simulink model "ChkPwrMding_newLogic"  (Simulink 7.8)
settings: Solver=ode45  StartTime=0.0  StopTime=10.0  RelTol=1e-3
undefined symbols (not defined in the file): CeSTMR_e_LVR_N, CeSTMR_e_LVR_P, KeASMR_b_CheckParkAndNeutral, KeASMR_b_StrtCntrlOffChkEnbl
libraries: ChryslerLib x2
settings Model: Creator=Ben  LastModifiedBy=Ben

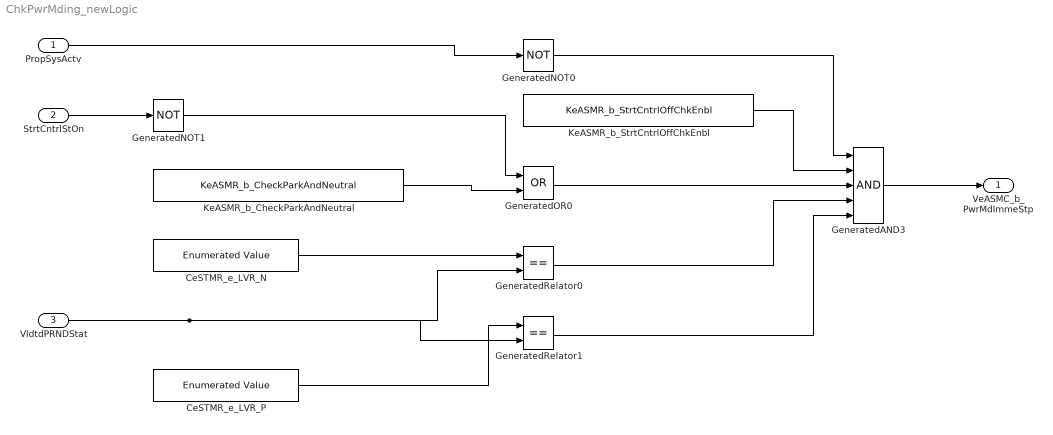
== system ChkPwrMding_newLogic ==
  PropSysActv : Inport
  StrtCntrlStOn : Inport  Port=2
  VldtdPRNDStat : Inport  Port=3
  CeSTMR_e_LVR_N : ChryslerLib/Parameters & Constants/Enumerated Value  Value=CeSTMR_e_LVR_N  OutMin=[]  OutMax=[]  OutDataTypeStr=TeSTMR_e_Lv2PRND_Stat
  CeSTMR_e_LVR_P : ChryslerLib/Parameters & Constants/Enumerated Value  Value=CeSTMR_e_LVR_P  OutMin=[]  OutMax=[]  OutDataTypeStr=TeSTMR_e_Lv2PRND_Stat
  GeneratedAND3 : Logic  Inputs=5
  GeneratedNOT0 : Logic  Operator=NOT
  GeneratedNOT1 : Logic  Operator=NOT
  GeneratedOR0 : Logic  Operator=OR
  GeneratedRelator0 : RelationalOperator  Operator===  InputSameDT=on
  GeneratedRelator1 : RelationalOperator  Operator===  InputSameDT=on
  KeASMR_b_CheckParkAndNeutral : Constant  Value=KeASMR_b_CheckParkAndNeutral
      settings: CopyFcn=try,set_param(gcb,'Value',get_param(gcb,'Name'));catch,err=lasterror;if (isempty(strfind(err.message,'Attempting to override parameters')) || isempty(strfind(err.message,'which is inside a library link'))) rethrow(err);end;end  NameChangeFcn=try,set_param(gcb,'Value',get_param(gcb,'Name'));catch,[msgstr msgid]=lasterr;errordlg(['error ',num2str(msgid),' - ',msgstr],'Error','modal');end  OpenFcn=global edelemcal; edelemcal.cb = gcb; edfigelemcal('fig');
  KeASMR_b_StrtCntrlOffChkEnbl : Constant  Value=KeASMR_b_StrtCntrlOffChkEnbl
      settings: CopyFcn=try,set_param(gcb,'Value',get_param(gcb,'Name'));catch,err=lasterror;if (isempty(strfind(err.message,'Attempting to override parameters')) || isempty(strfind(err.message,'which is inside a library link'))) rethrow(err);end;end  NameChangeFcn=try,set_param(gcb,'Value',get_param(gcb,'Name'));catch,[msgstr msgid]=lasterr;errordlg(['error ',num2str(msgid),' - ',msgstr],'Error','modal');end  OpenFcn=global edelemcal; edelemcal.cb = gcb; edfigelemcal('fig');
  VeASMC_b_PwrMdImmeStp : Outport
  wires:
  VldtdPRNDStat/1 -> GeneratedRelator0/2, GeneratedRelator1/2
  GeneratedNOT0/1 -> GeneratedAND3/1
  KeASMR_b_StrtCntrlOffChkEnbl/1 -> GeneratedAND3/2
  GeneratedOR0/1 -> GeneratedAND3/3
  GeneratedRelator0/1 -> GeneratedAND3/4
  GeneratedRelator1/1 -> GeneratedAND3/5
  PropSysActv/1 -> GeneratedNOT0/1
  StrtCntrlStOn/1 -> GeneratedNOT1/1
  GeneratedNOT1/1 -> GeneratedOR0/1
  KeASMR_b_CheckParkAndNeutral/1 -> GeneratedOR0/2
  CeSTMR_e_LVR_N/1 -> GeneratedRelator0/1
  CeSTMR_e_LVR_P/1 -> GeneratedRelator1/1
  GeneratedAND3/1 -> VeASMC_b_PwrMdImmeStp/1
